simulink model "PIDVER2"  (R2013b)
settings: Solver=FixedStepDiscrete  SolverMode=SingleTasking  StartTime=0.0  StopTime=1000  FixedStep=1  RelTol=1e-3
libraries: xbsIndex_r4 x29, simulink x5
settings Model: Creator=laca  LastModifiedBy=laca

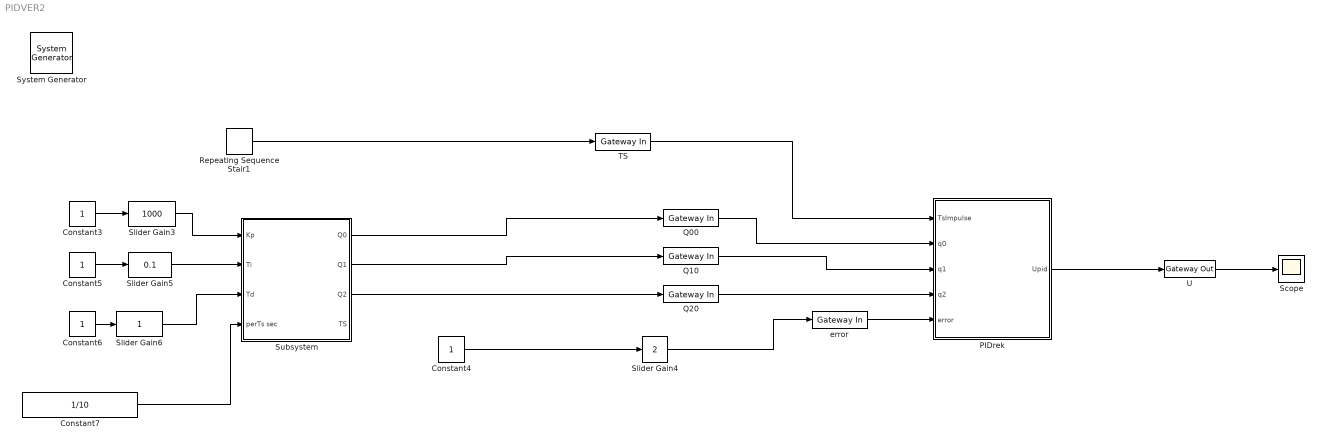
== system PIDVER2 ==
  " System Generator" : xbsIndex_r4/ System Generator  Tag=genX  xilinxfamily=spartan3e  part=xc3s500e  speed=-4  package=pq208  synthesis_tool=XST  clock_wrapper=Clock Enables  directory=./netlist  proj_type=Project Navigator  Synth_file=XST Defaults  Impl_file=ISE Defaults  testbench=off  simulink_period=1  sysclk_period=20  dcm_input_clock_period=10  incr_netlist=off  trim_vbits=Everywhere in SubSystem  dbl_ovrd=According to Block Masks  core_generation=According to Block Masks  run_coregen=off  deprecated_control=off  eval_field=0  block_type=sysgen
  Constant{3..6} (4 alike) : Constant
  Constant7 : Constant  Value=1/10
  PIDrek : Subsystem
  Q00 : xbsIndex_r4/Gateway In  gui_display_data_type=Fixed-point  arith_type="Signed  (2's comp)"  n_bits=16  bin_pt=0  preci_type=Single  exp_width=8  frac_width=24  quantization="Round  (unbiased: +/- Inf)"  overflow=Saturate  period=1  dbl_ovrd=off  timing_constraint=None  locs_specified=off  LOCs={}  UseAsADC=off  ADCChannel='1'  inherit_from_input=off  hdl_port=on  block_type=gatewayin
  Q10 : xbsIndex_r4/Gateway In  gui_display_data_type=Fixed-point  arith_type="Signed  (2's comp)"  n_bits=16  bin_pt=0  preci_type=Single  exp_width=8  frac_width=24  quantization="Round  (unbiased: +/- Inf)"  overflow=Saturate  period=1  dbl_ovrd=off  timing_constraint=None  locs_specified=off  LOCs={}  UseAsADC=off  ADCChannel='1'  inherit_from_input=off  hdl_port=on  block_type=gatewayin
  Q20 : xbsIndex_r4/Gateway In  gui_display_data_type=Fixed-point  arith_type="Signed  (2's comp)"  n_bits=16  bin_pt=0  preci_type=Single  exp_width=8  frac_width=24  quantization="Round  (unbiased: +/- Inf)"  overflow=Saturate  period=1  dbl_ovrd=off  timing_constraint=None  locs_specified=off  LOCs={}  UseAsADC=off  ADCChannel='1'  inherit_from_input=off  hdl_port=on  block_type=gatewayin
  Repeating Sequence Stair1 : simulink/Sources/Repeating Sequence Stair  OutValues=[0 1 0 0 0 0 0 0 0 0 0 0 0 0 0 0 0 0 0 0 ].'  tsamp=1  OutMin=[]  OutMax=[]  OutDataTypeStr=double  OutputDataTypeScalingMode=double  OutDataType=fixdt(0,8)  ConRadixGroup=Best Precision: Vector-wise  OutScaling=2^-12
  Scope : Scope
  Slider Gain3 : simulink/Math Operations/Slider Gain  low=0  gain=1000  high=65000
  Slider Gain4 : simulink/Math Operations/Slider Gain  low=0  gain=2  high=50000
  Slider Gain5 : simulink/Math Operations/Slider Gain  low=0  gain=0.1  high=65000
  Slider Gain6 : simulink/Math Operations/Slider Gain  low=0  gain=1  high=5000
  Subsystem : Subsystem
  TS : xbsIndex_r4/Gateway In  gui_display_data_type=Boolean  arith_type=Boolean  n_bits=16  bin_pt=0  preci_type=Single  exp_width=8  frac_width=24  quantization="Round  (unbiased: +/- Inf)"  overflow=Saturate  period=1  dbl_ovrd=off  timing_constraint=None  locs_specified=off  LOCs={}  UseAsADC=off  ADCChannel='1'  inherit_from_input=off  hdl_port=on  block_type=gatewayin
  U : xbsIndex_r4/Gateway Out  inherit_from_input=off  hdl_port=on  timing_constraint=None  locs_specified=off  LOCs={}  UseAsDAC=off  DACChannel='1'  block_type=gatewayout
  error : xbsIndex_r4/Gateway In  gui_display_data_type=Fixed-point  arith_type=Unsigned  n_bits=16  bin_pt=0  preci_type=Single  exp_width=8  frac_width=24  quantization="Round  (unbiased: +/- Inf)"  overflow=Saturate  period=1  dbl_ovrd=off  timing_constraint=None  locs_specified=off  LOCs={}  UseAsADC=off  ADCChannel='1'  inherit_from_input=off  hdl_port=on  block_type=gatewayin
  wires:
  TS/1 -> PIDrek/1(TsImpulse)
  Repeating Sequence Stair1/1 -> TS/1
  Constant4/1 -> Slider Gain4/1
  Slider Gain4/1 -> error/1
  Q00/1 -> PIDrek/2(q0)
  Q10/1 -> PIDrek/3(q1)
  Q20/1 -> PIDrek/4(q2)
  error/1 -> PIDrek/5(error)
  Constant3/1 -> Slider Gain3/1
  Constant5/1 -> Slider Gain5/1
  Constant6/1 -> Slider Gain6/1
  Slider Gain3/1 -> Subsystem/1(Kp)
  Slider Gain5/1 -> Subsystem/2(Ti)
  Slider Gain6/1 -> Subsystem/3(Td)
  Constant7/1 -> Subsystem/4(perTs sec)
  Subsystem/1(Q0) -> Q00/1
  Subsystem/2(Q1) -> Q10/1
  Subsystem/3(Q2) -> Q20/1
  U/1 -> Scope/1
  PIDrek/1(Upid) -> U/1

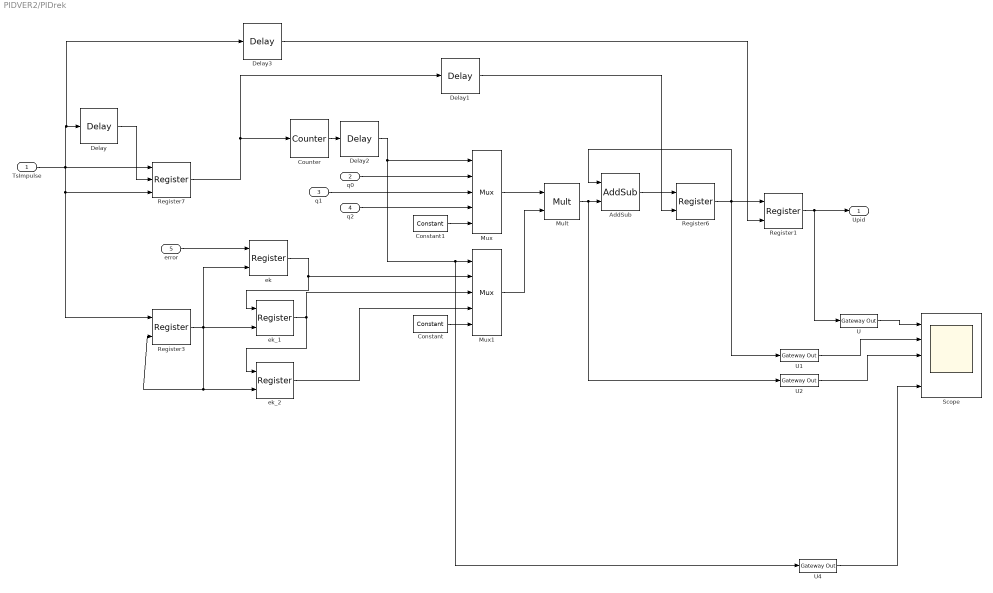
== system PIDVER2/PIDrek ==
  TsImpulse : Inport
  q0 : Inport  Port=2
  q1 : Inport  Port=3
  q2 : Inport  Port=4
  error : Inport  Port=5
  AddSub : xbsIndex_r4/AddSub  mode=Addition  use_carryin=off  use_carryout=off  en=off  latency=0  precision=User Defined  arith_type="Signed  (2's comp)"  n_bits=17  bin_pt=0  quantization=Truncate  overflow=Saturate  dbl_ovrd=off  use_behavioral_HDL=off  hw_selection=Fabric  pipelined=off  block_type=addsub
  Constant : xbsIndex_r4/Constant  const=0  gui_display_data_type=Fixed-point  arith_type=Signed (2's comp)  n_bits=16  bin_pt=0  preci_type=Single  exp_width=8  frac_width=24  explicit_period=off  period=1  equ=P=C  opselect=C  inp2=PCIN>>17  opr=+  inp1=P  carry=CIN  dbl_ovrd=off  block_type=constant
  Constant1 : xbsIndex_r4/Constant  const=0  gui_display_data_type=Fixed-point  arith_type=Signed (2's comp)  n_bits=16  bin_pt=0  preci_type=Single  exp_width=8  frac_width=24  explicit_period=off  period=1  equ=P=C  opselect=C  inp2=PCIN>>17  opr=+  inp1=P  carry=CIN  dbl_ovrd=off  block_type=constant
  Counter : xbsIndex_r4/Counter  cnt_type=Count Limited  cnt_to=2  operation=Up  start_count=0  cnt_by_val=1  arith_type=Unsigned  n_bits=2  bin_pt=0  load_pin=off  rst=off  en=on  explicit_period=on  period=1  dbl_ovrd=off  use_behavioral_HDL=off  implementation=Fabric  block_type=counter
  Delay : xbsIndex_r4/Delay  rst=off  infoeditControl=Selection of Reset will increase slice count due to use of real FFs and instead of SRLs  en=off  latency=3  dbl_ovrd=off  reg_retiming=off  block_type=delay
  Delay1 : xbsIndex_r4/Delay  rst=off  infoeditControl=Selection of Reset will increase slice count due to use of real FFs and instead of SRLs  en=off  latency=2  dbl_ovrd=off  reg_retiming=off  block_type=delay
  Delay2 : xbsIndex_r4/Delay  rst=off  infoeditControl=Selection of Reset will increase slice count due to use of real FFs and instead of SRLs  en=off  latency=1  dbl_ovrd=off  reg_retiming=off  block_type=delay
  Delay3 : xbsIndex_r4/Delay  rst=off  infoeditControl=Selection of Reset will increase slice count due to use of real FFs and instead of SRLs  en=off  latency=4  dbl_ovrd=off  reg_retiming=off  block_type=delay
  Mult : xbsIndex_r4/Mult  precision=User Defined  arith_type="Signed  (2's comp)"  n_bits=17  bin_pt=0  quantization=Truncate  overflow=Saturate  en=off  latency=1  dbl_ovrd=off  use_behavioral_HDL=off  opt=Speed  use_embedded=on  optimum_pipeline=off  pipeline=on  use_rpm=on  placement_style=Triangular  block_type=mult
  Mux : xbsIndex_r4/Mux  inputs=4  en=off  latency=0  precision=User Defined  arith_type="Signed  (2's comp)"  n_bits=16  bin_pt=0  quantization=Truncate  overflow=Saturate  dbl_ovrd=off  block_type=mux
  Mux1 : xbsIndex_r4/Mux  inputs=4  en=off  latency=0  precision=User Defined  arith_type="Signed  (2's comp)"  n_bits=16  bin_pt=0  quantization=Truncate  overflow=Saturate  dbl_ovrd=off  block_type=mux
  Register1 : xbsIndex_r4/Register  init=0  rst=off  en=on  dbl_ovrd=off  block_type=register
  Register3 : xbsIndex_r4/Register  init=0  rst=on  en=off  dbl_ovrd=off  block_type=register
  Register6 : xbsIndex_r4/Register  init=0  rst=off  en=on  dbl_ovrd=off  block_type=register
  Register7 : xbsIndex_r4/Register  init=0  rst=on  en=on  dbl_ovrd=off  block_type=register
  Scope : Scope  NumInputPorts=5
      settings: TimeRange=1000  YMin=-5~-5~-5~-5~-5  YMax=5~5~5~5~5  SaveName=ScopeData2
  U{,1..2,4} (4 alike) : xbsIndex_r4/Gateway Out  inherit_from_input=off  hdl_port=on  timing_constraint=None  locs_specified=off  LOCs={}  UseAsDAC=off  DACChannel='1'  block_type=gatewayout
  ek : xbsIndex_r4/Register  init=0  rst=off  en=on  dbl_ovrd=off  block_type=register
  ek_1 : xbsIndex_r4/Register  init=0  rst=off  en=on  dbl_ovrd=off  block_type=register
  ek_2 : xbsIndex_r4/Register  init=0  rst=off  en=on  dbl_ovrd=off  block_type=register
  Upid : Outport
  wires:
  Mux/1 -> Mult/1
  Mux1/1 -> Mult/2
  q0/1 -> Mux/2
  ek/1 -> Mux1/2, ek_1/1
  ek_1/1 -> Mux1/3, ek_2/1
  AddSub/1 -> Register6/1
  error/1 -> ek/1
  Delay/1 -> Register7/2
  Register3/1 -> Register3/2, ek_2/2, ek_1/2, ek/2
  Counter/1 -> Delay2/1
  Delay1/1 -> Register6/2
  Delay2/1 -> U4/1, Mux1/1, Mux/1
  TsImpulse/1 -> Register3/1, Register7/3, Delay3/1, Delay/1, Register7/1
  Constant/1 -> Mux1/5
  Register7/1 -> Delay1/1, Counter/1
  Constant1/1 -> Mux/5
  q1/1 -> Mux/3
  q2/1 -> Mux/4
  ek_2/1 -> Mux1/4
  U/1 -> Scope/1
  U1/1 -> Scope/2
  Mult/1 -> U2/1, AddSub/2
  U2/1 -> Scope/3
  ? -> Scope/4
  U4/1 -> Scope/5
  Register6/1 -> U1/1, Register1/1, AddSub/1
  Register1/1 -> U/1, Upid/1
  Delay3/1 -> Register1/2

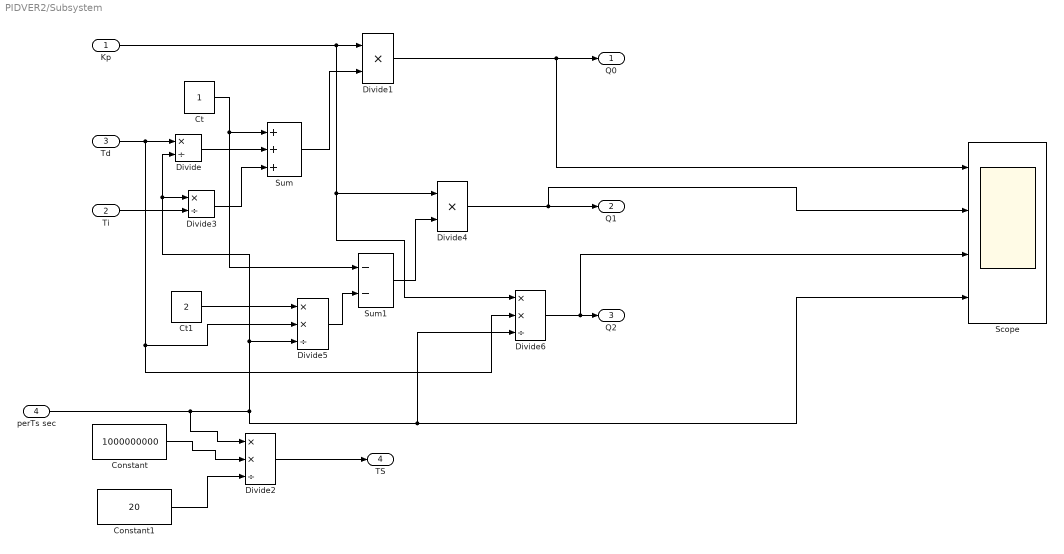
== system PIDVER2/Subsystem ==
  Kp : Inport
  Ti : Inport  Port=2
  Td : Inport  Port=3
  perTs sec : Inport  Port=4
  Constant : Constant  Value=1000000000
  Constant1 : Constant  Value=20
  Ct : Constant
  Ct1 : Constant  Value=2
  Divide : Product  Inputs=*/
  Divide1 : Product  Inputs=**
  Divide2 : Product  Inputs=**/
  Divide3 : Product  Inputs=*/
  Divide4 : Product  Inputs=**
  Divide5 : Product  Inputs=**/
  Divide6 : Product  Inputs=**/
  Scope : Scope  NumInputPorts=4
      settings: TimeRange=1000  YMin=1.3659~1.7179~2375~237.5  YMax=1.50968~1.89874~2625~262.5
  Sum : Sum  Inputs=+++
  Sum1 : Sum  Inputs=--
  Q0 : Outport
  Q1 : Outport  Port=2
  Q2 : Outport  Port=3
  TS : Outport  Port=4
  wires:
  perTs sec/1 -> Divide2/1, Scope/4, Divide6/3, Divide5/3, Divide3/1, Divide/2
  Constant/1 -> Divide2/2
  Constant1/1 -> Divide2/3
  Kp/1 -> Divide6/1, Divide4/1, Divide1/1
  Ct/1 -> Sum1/1, Sum/1
  Divide/1 -> Sum/2
  Td/1 -> Divide6/2, Divide5/2, Divide/1
  Ti/1 -> Divide3/2
  Divide3/1 -> Sum/3
  Sum/1 -> Divide1/2
  Divide1/1 -> Scope/1, Q0/1
  Divide4/1 -> Scope/2, Q1/1
  Sum1/1 -> Divide4/2
  Divide5/1 -> Sum1/2
  Ct1/1 -> Divide5/1
  Divide6/1 -> Scope/3, Q2/1
  Divide2/1 -> TS/1
